simulink model "Exercise11_2"  (R2018b)
settings: Solver=VariableStepAuto  StartTime=0.0  StopTime=10.0  RelTol=1e-3
settings Model: Creator=Ramiro  LastModifiedBy=Ramiro

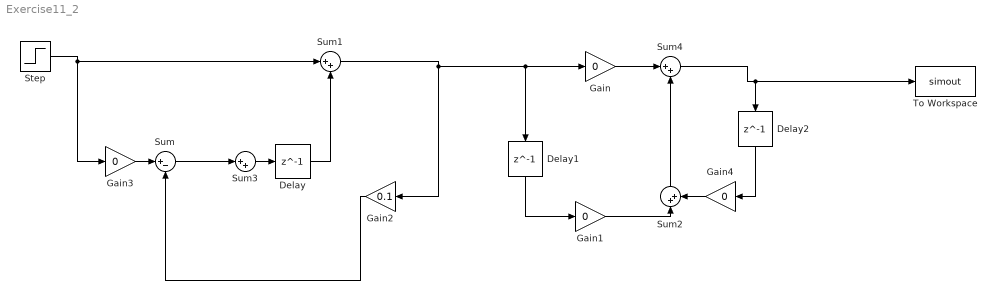
== system Exercise11_2 ==
  Delay : Delay  DelayLength=1  InitialCondition=0
  Delay1 : Delay  DelayLength=1  InitialCondition=0
  Delay2 : Delay  DelayLength=1  InitialCondition=0
  Gain{,1,3..4} (4 alike) : Gain  Gain=0
  Gain2 : Gain  Gain=0.1
  Step : Step  SampleTime=0
  Sum : Sum  Inputs=|+-
  Sum{1..4} (4 alike) : Sum  Inputs=|++
  To Workspace : ToWorkspace  VariableName=simout  SaveFormat=Timeseries  SampleTime=-1
  wires:
  Sum1/1 -> Delay1/1, Gain/1, Gain2/1
  Gain2/1 -> Sum/2
  Gain3/1 -> Sum/1
  Step/1 -> Sum1/1, Gain3/1
  Sum/1 -> Sum3/1
  Sum3/1 -> Delay/1
  Delay/1 -> Sum1/2
  Gain/1 -> Sum4/1
  Sum4/1 -> Delay2/1, To Workspace/1
  Delay2/1 -> Gain4/1
  Delay1/1 -> Gain1/1
  Sum2/1 -> Sum4/2
  Gain1/1 -> Sum2/1
  Gain4/1 -> Sum2/2
